simulink model "Lab02_Part3"  (R2017b)
settings: Solver=VariableStepAuto  StartTime=0.0  StopTime=tf  MaxStep=maxstep  RelTol=tol  AbsTol=tol
values from neighbouring files (symbols this model uses):
  b = 1    [Lab2Script.m]    (also in Lab2Script_class.m)
  force = 6    [Lab2Script.m]
  k = 20    [Lab2Script.m]
  m = 2    [Lab2Script.m]    (also in Lab2Script_class.m = 1)
  x0 = 0.2    [Lab2Script.m]
  xdot0 = -1    [Lab2Script.m]
settings Model: Creator=rodrigue  LastModifiedBy=rodrigue

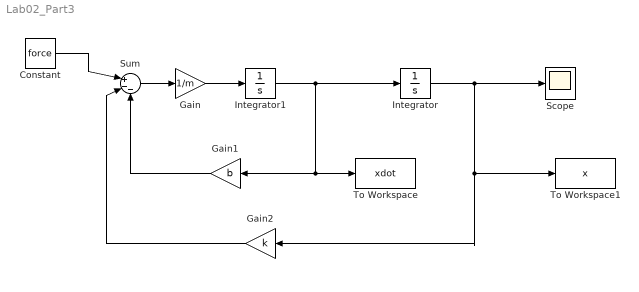
== system Lab02_Part3 ==
  Constant : Constant  Value=force
  Gain : Gain  Gain=1/m
  Gain1 : Gain  Gain=b
  Gain2 : Gain  Gain=k
  Integrator : Integrator  InitialCondition=x0
  Integrator1 : Integrator  InitialCondition=xdot0
  Scope : Scope
  Sum : Sum  Inputs=|+--
  To Workspace : ToWorkspace  VariableName=xdot  SampleTime=-1
  To Workspace1 : ToWorkspace  VariableName=x  SampleTime=-1
  wires:
  Constant/1 -> Sum/1
  Sum/1 -> Gain/1
  Gain/1 -> Integrator1/1
  Integrator1/1 -> Gain1/1, To Workspace/1, Integrator/1
  Gain1/1 -> Sum/3
  Integrator/1 -> To Workspace1/1, Gain2/1, Scope/1
  Gain2/1 -> Sum/2
